simulink model "MGDC_RL"  (R2025b)
settings: Solver=VariableStepAuto  StartTime=0.0  StopTime=12  RelTol=1e-3
libraries: spsGroundLib x8, spsControlledVoltageSourceLib x3, spsCurrentMeasurementLib x3, spsParallelRLCBranchLib x3, spsVoltageMeasurementLib x3, spsSeriesRLCBranchLib x2, spsBreakerLib x1, sps_lib x1
(part 1 of 4)
settings Model: Creator=joseA  LastModifiedBy=joseA

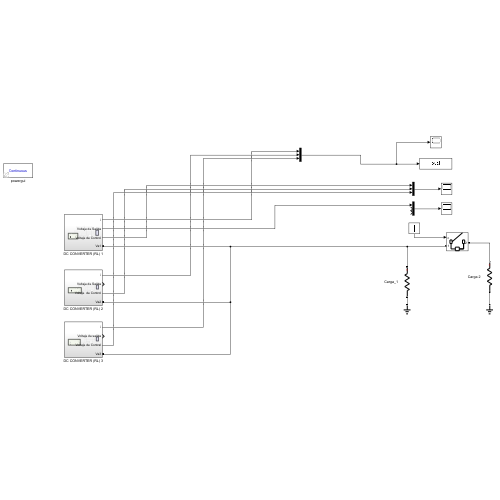
[thumbnail: Simulink's stored preview of the top-level diagram]
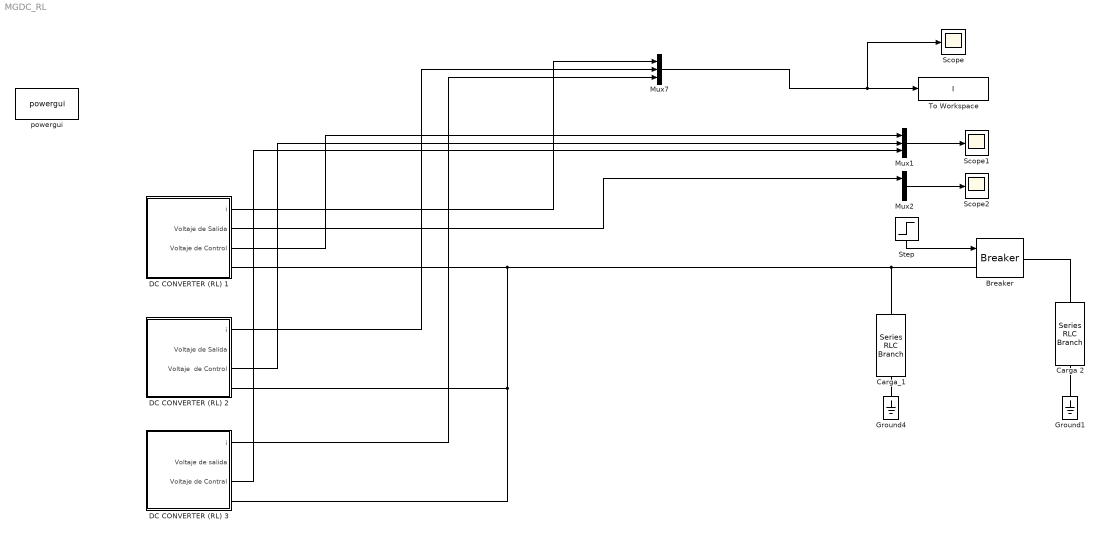
== system MGDC_RL ==
  Breaker : spsBreakerLib/Breaker  InitialState=0  SwitchingTimes="[1/60  5/60]"  External=on  BreakerResistance=0.01  SnubberResistance=1e6  SnubberCapacitance=inf  Measurements=None  MoreParameters=on  NoBreakLoop=off
  Carga 2 : spsSeriesRLCBranchLib/Series RLC Branch  LConnTagsString=__new0  RConnTagsString=__new0  BranchType=R  Resistance=4  Inductance=1e-3  SetiL0=off  InitialCurrent=0  Capacitance=1e-6  Setx0=off  InitialVoltage=0  Measurements=None
  Carga_1 : spsSeriesRLCBranchLib/Series RLC Branch  LConnTagsString=__new0  RConnTagsString=__new0  BranchType=R  Resistance=8  Inductance=1e-3  SetiL0=off  InitialCurrent=0  Capacitance=1e-6  Setx0=off  InitialVoltage=0  Measurements=None
  DC CONVERTER (RL) 1 : Subsystem
      settings: PortSchema="{\"entries\":[{\"content\":{\"sides\":[{\"content\":{\"connectorIds\":[\"Out1\",\"Out2\",\"Out3\",\"LConn1\"]},\"type\":\"ConnectorPlacement.EquallySpacedRectSide\",\"uuid\":\"ef85fad9-e9fc-446c-84f1-0628c69dc682\"},{\"content\":{\"side\":\"RIGHT\"},\"type\":\"ConnectorPlacement.EquallySpacedRectSide\",\"uuid\":\"b40e7fcd-3dee-4863-8a64-1e7c5a18af7f\"},{\"content\":{\"side\":\"TOP\"},\"type\":\"ConnectorPlacement.EquallySpacedRectSide\",\"uuid\":\"d80d7a5f-fa61-4dc2-bf12-1a6ce1f92f0b\"}]},\"type\":\"ConnectorPlacement.EquallySpacedConnector\",\"uuid\":\"ea08e065-469c-42e9-9976-17e3ee08db16\"}],\"packageUris\":[\"http://schema.mathworks.com/mf0/Connector/R2020b\"],\"version\":\"1.0\"}"
  DC CONVERTER (RL) 2 : Subsystem
      settings: PortSchema="{\"entries\":[{\"content\":{\"sides\":[{\"content\":{\"connectorIds\":[\"Out1\",\"Out2\",\"Out3\",\"LConn1\"]},\"type\":\"ConnectorPlacement.EquallySpacedRectSide\",\"uuid\":\"ef85fad9-e9fc-446c-84f1-0628c69dc682\"},{\"content\":{\"side\":\"RIGHT\"},\"type\":\"ConnectorPlacement.EquallySpacedRectSide\",\"uuid\":\"b40e7fcd-3dee-4863-8a64-1e7c5a18af7f\"},{\"content\":{\"side\":\"TOP\"},\"type\":\"ConnectorPlacement.EquallySpacedRectSide\",\"uuid\":\"d80d7a5f-fa61-4dc2-bf12-1a6ce1f92f0b\"}]},\"type\":\"ConnectorPlacement.EquallySpacedConnector\",\"uuid\":\"ea08e065-469c-42e9-9976-17e3ee08db16\"}],\"packageUris\":[\"http://schema.mathworks.com/mf0/Connector/R2020b\"],\"version\":\"1.0\"}"
  DC CONVERTER (RL) 3 : Subsystem
      settings: PortSchema="{\"entries\":[{\"content\":{\"sides\":[{\"content\":{\"connectorIds\":[\"Out1\",\"Out2\",\"Out3\",\"LConn1\"]},\"type\":\"ConnectorPlacement.EquallySpacedRectSide\",\"uuid\":\"ef85fad9-e9fc-446c-84f1-0628c69dc682\"},{\"content\":{\"side\":\"RIGHT\"},\"type\":\"ConnectorPlacement.EquallySpacedRectSide\",\"uuid\":\"b40e7fcd-3dee-4863-8a64-1e7c5a18af7f\"},{\"content\":{\"side\":\"TOP\"},\"type\":\"ConnectorPlacement.EquallySpacedRectSide\",\"uuid\":\"d80d7a5f-fa61-4dc2-bf12-1a6ce1f92f0b\"}]},\"type\":\"ConnectorPlacement.EquallySpacedConnector\",\"uuid\":\"ea08e065-469c-42e9-9976-17e3ee08db16\"}],\"packageUris\":[\"http://schema.mathworks.com/mf0/Connector/R2020b\"],\"version\":\"1.0\"}"
  Ground1 : spsGroundLib/Ground  LConnTagsString=a
  Ground4 : spsGroundLib/Ground  LConnTagsString=a
  Mux1 : Mux  Inputs=3
  Mux2 : Mux  Inputs=3
  Mux7 : Mux  Inputs=3
  Scope : Scope
      settings: ActiveDisplayYMinimum=-0.5913391401684992  ActiveDisplayYMaximum=5.3220510444351152
  Scope1 : Scope
      settings: ActiveDisplayYMinimum=-0.069374999999999867  ActiveDisplayYMaximum=0.67437499999999884
  Scope2 : Scope
      settings: ActiveDisplayYMinimum=-3.0088602206152393  ActiveDisplayYMaximum=27.079741985537161  DataLoggingVariableName=ScopeData3
  Step : Step  Time=6.5  SampleTime=0
  To Workspace : ToWorkspace  VariableName=I  SaveFormat=Timeseries  SampleTime=-1
  powergui : sps_lib/powergui  Priority=1  SimulationMode=Continuous  SampleTime=50e-6  frequency=60  Iterations=50  frequencyindice=0  Pbase=100e6  ErrMax=1e-4  UnitsV=kV  UnitsW=MW  buscounter=0  FunctionMessages=off  echomessages=off  EnableUseOfTLC=off  CurrentSourceSwitches=off  DisableSnubberDevices=off  DisableRonSwitches=off  DisableVfSwitches=off  DisplayEquations=off  AutomaticDiscreteSolvers=off  SolverType=Tustin/Backward Euler (TBE)  Interpol=off  ExternalGateDelay=off  methode=off  Ts=100  x0status=blocks  SPID=on  SwTol=0  HookPort=off  NonlinearTolerance=1e-4  nMaxIteration=100  ContinueOnMaxIteration=off  RestoreLinks=warning  ResistiveCurrentMeasurement=off  Frange=[0:2:500]  Ylog=off  Xlog=on  ShowGrid=off  save=off  variable=ZData  structure=0  ZoomFFT=off  StartTime=0.0  cycles=1  DisplayStyle=1  fundamental=60  FreqAxis=off  MaxFrequency=1000  frequencyindicesteady=1  RmsSteady=1  display=off
  wires:
  Step/1 -> Breaker/1
  DC CONVERTER (RL) 1/1(i) -> Mux7/1
  DC CONVERTER (RL) 3/1(i) -> Mux7/3
  Mux7/1 -> Scope/1, To Workspace/1
  DC CONVERTER (RL) 2/1(i) -> Mux7/2
  DC CONVERTER (RL) 1/3(Voltaje de Control) -> Mux1/1
  Mux1/1 -> Scope1/1
  DC CONVERTER (RL) 2/3(Voltaje  de Control) -> Mux1/2
  DC CONVERTER (RL) 3/3(Voltaje de Contral) -> Mux1/3
  DC CONVERTER (RL) 1/2(Voltaje de Salida) -> Mux2/1
  Mux2/1 -> Scope2/1
  connections:
  Ground1/LConn1 -- Carga 2/RConn1
  Ground4/LConn1 -- Carga_1/RConn1
  Carga 2/LConn1 -- Breaker/RConn1
  DC CONVERTER (RL) 2/LConn1 -- DC CONVERTER (RL) 3/LConn1 -- Breaker/LConn1 -- Carga_1/LConn1 -- DC CONVERTER (RL) 1/LConn1

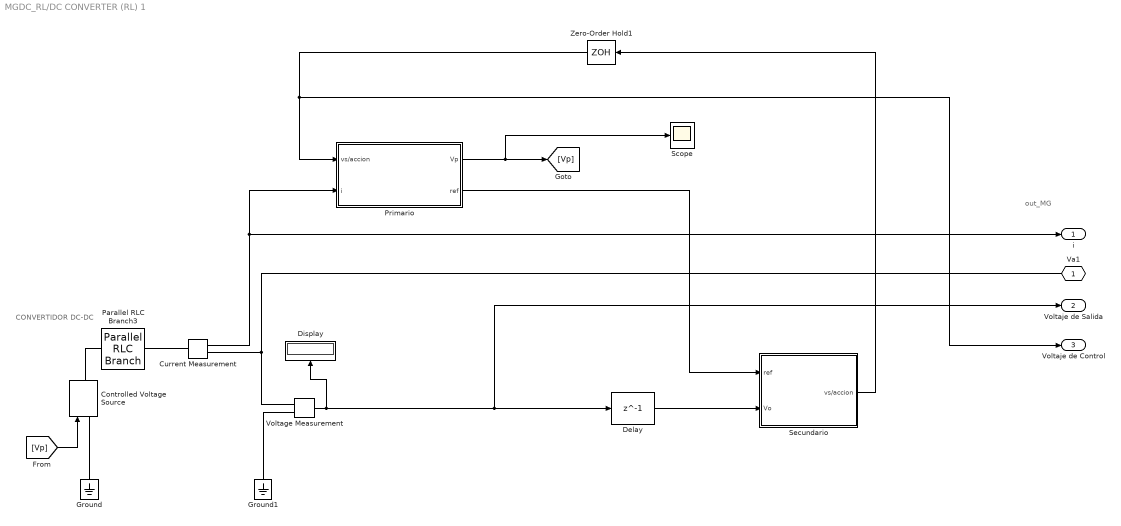
== system MGDC_RL/DC CONVERTER (RL) 1 ==
  note: out_MG
  note: CONVERTIDOR DC-DC
  Controlled Voltage Source : spsControlledVoltageSourceLib/Controlled Voltage Source  Initialize=on  Source_Type=DC  Amplitude=0  Phase=0  Frequency=0  Measurements=None
  Current Measurement : spsCurrentMeasurementLib/Current Measurement  PhasorSimulation=off  OutputType=Complex  PSBequivalent=0
  Delay : Delay  DelayLength=1  InitialCondition=0  UseCircularBuffer=on
  Display : Display
  Ground : spsGroundLib/Ground  LConnTagsString=a
  Ground1 : spsGroundLib/Ground  LConnTagsString=a
  Parallel RLC Branch3 : spsParallelRLCBranchLib/Parallel RLC Branch  LConnTagsString=a  RConnTagsString=__new0  BranchType=R  Resistance=0.01  Inductance=1e-3  SetiL0=off  InitialCurrent=0  Capacitance=1e-6  Setx0=off  InitialVoltage=0  Measurements=None
  Primario : Subsystem
  Scope : Scope
      settings: ActiveDisplayYMinimum=-1  ActiveDisplayYMaximum=1  DataLoggingVariableName=ScopeData2
  "Secundario " : Subsystem
  Voltage Measurement : spsVoltageMeasurementLib/Voltage Measurement  PhasorSimulation=off  OutputType=Complex  PSBequivalent=0
  Zero-Order Hold1 : ZeroOrderHold  SampleTime=0.01
  Va1 : PMIOPort  Tag=PMCPort  Side=Left
  i : Outport
  Voltaje de Salida : Outport  Port=2
  Voltaje de Control : Outport  Port=3
  wires:
  Voltage Measurement/1 -> Voltaje de Salida/1, Delay/1, Display/1
  [Vp] -> Controlled Voltage Source/1
  Zero-Order Hold1/1 -> Primario/1(vs/accion), Voltaje de Control/1
  Current Measurement/1 -> i/1, Primario/2(i)
  "Secundario "/1(vs/accion) -> Zero-Order Hold1/1
  Primario/2(ref) -> "Secundario "/1(ref)
  Delay/1 -> "Secundario "/2(Vo)
  Primario/1(Vp) -> Scope/1, [Vp]
  connections:
  Voltage Measurement/LConn2 -- Ground1/LConn1
  Ground/LConn1 -- Controlled Voltage Source/LConn1
  Parallel RLC Branch3/LConn1 -- Current Measurement/LConn1
  Voltage Measurement/LConn1 -- Va1/RConn1 -- Current Measurement/RConn1
  Controlled Voltage Source/RConn1 -- Parallel RLC Branch3/RConn1

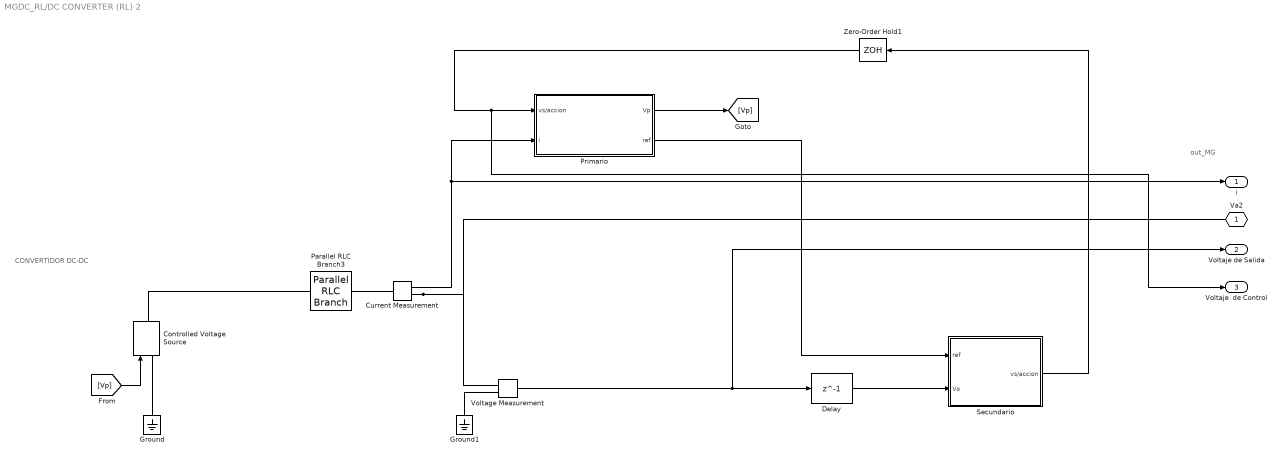
== system MGDC_RL/DC CONVERTER (RL) 2 ==
  note: out_MG
  note: CONVERTIDOR DC-DC
  Controlled Voltage Source : spsControlledVoltageSourceLib/Controlled Voltage Source  Initialize=on  Source_Type=DC  Amplitude=0  Phase=0  Frequency=0  Measurements=None
  Current Measurement : spsCurrentMeasurementLib/Current Measurement  PhasorSimulation=off  OutputType=Complex  PSBequivalent=0
  Delay : Delay  DelayLength=1  InitialCondition=0  UseCircularBuffer=on
  Ground : spsGroundLib/Ground  LConnTagsString=a
  Ground1 : spsGroundLib/Ground  LConnTagsString=a
  Parallel RLC Branch3 : spsParallelRLCBranchLib/Parallel RLC Branch  LConnTagsString=a  RConnTagsString=__new0  BranchType=R  Resistance=0.01  Inductance=1e-3  SetiL0=off  InitialCurrent=0  Capacitance=1e-6  Setx0=off  InitialVoltage=0  Measurements=None
  Primario : Subsystem
  "Secundario " : Subsystem
  Voltage Measurement : spsVoltageMeasurementLib/Voltage Measurement  PhasorSimulation=off  OutputType=Complex  PSBequivalent=0
  Zero-Order Hold1 : ZeroOrderHold  SampleTime=0.01
  Va2 : PMIOPort  Tag=PMCPort  Side=Left
  i : Outport
  Voltaje de Salida : Outport  Port=2
  Voltaje  de Control : Outport  Port=3
  wires:
  Voltage Measurement/1 -> Voltaje de Salida/1, Delay/1
  [Vp] -> Controlled Voltage Source/1
  Zero-Order Hold1/1 -> Voltaje  de Control/1, Primario/1(vs/accion)
  Current Measurement/1 -> i/1, Primario/2(i)
  "Secundario "/1(vs/accion) -> Zero-Order Hold1/1
  Primario/2(ref) -> "Secundario "/1(ref)
  Primario/1(Vp) -> [Vp]
  Delay/1 -> "Secundario "/2(Vo)
  connections:
  Voltage Measurement/LConn2 -- Ground1/LConn1
  Ground/LConn1 -- Controlled Voltage Source/LConn1
  Current Measurement/LConn1 -- Parallel RLC Branch3/LConn1
  Current Measurement/RConn1 -- Voltage Measurement/LConn1 -- Va2/RConn1
  Controlled Voltage Source/RConn1 -- Parallel RLC Branch3/RConn1

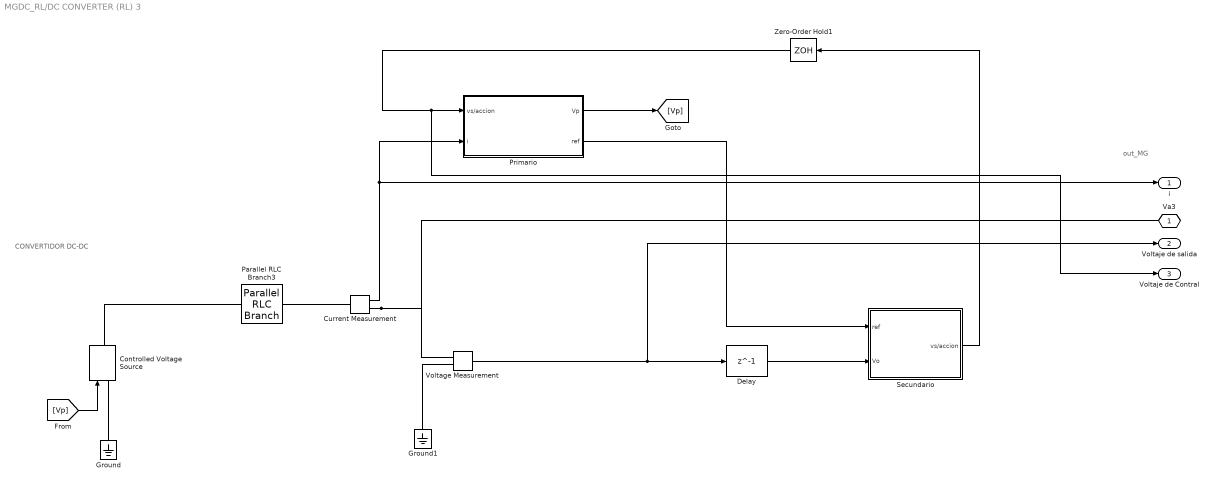
== system MGDC_RL/DC CONVERTER (RL) 3 ==
  note: out_MG
  note: CONVERTIDOR DC-DC
  Controlled Voltage Source : spsControlledVoltageSourceLib/Controlled Voltage Source  Initialize=on  Source_Type=DC  Amplitude=0  Phase=0  Frequency=0  Measurements=None
  Current Measurement : spsCurrentMeasurementLib/Current Measurement  PhasorSimulation=off  OutputType=Complex  PSBequivalent=0
  Delay : Delay  DelayLength=1  InitialCondition=0  UseCircularBuffer=on
  Ground : spsGroundLib/Ground  LConnTagsString=a
  Ground1 : spsGroundLib/Ground  LConnTagsString=a
  Parallel RLC Branch3 : spsParallelRLCBranchLib/Parallel RLC Branch  LConnTagsString=a  RConnTagsString=__new0  BranchType=R  Resistance=0.01  Inductance=1e-3  SetiL0=off  InitialCurrent=0  Capacitance=1e-6  Setx0=off  InitialVoltage=0  Measurements=None
  Primario : Subsystem
  "Secundario " : Subsystem
  Voltage Measurement : spsVoltageMeasurementLib/Voltage Measurement  PhasorSimulation=off  OutputType=Complex  PSBequivalent=0
  Zero-Order Hold1 : ZeroOrderHold  SampleTime=0.01
  Va3 : PMIOPort  Tag=PMCPort  Side=Left
  i : Outport
  Voltaje de salida : Outport  Port=2
  Voltaje de Contral : Outport  Port=3
  wires:
  Voltage Measurement/1 -> Voltaje de salida/1, Delay/1
  [Vp] -> Controlled Voltage Source/1
  Zero-Order Hold1/1 -> Voltaje de Contral/1, Primario/1(vs/accion)
  Current Measurement/1 -> i/1, Primario/2(i)
  "Secundario "/1(vs/accion) -> Zero-Order Hold1/1
  Primario/2(ref) -> "Secundario "/1(ref)
  Delay/1 -> "Secundario "/2(Vo)
  Primario/1(Vp) -> [Vp]
  connections:
  Voltage Measurement/LConn2 -- Ground1/LConn1
  Ground/LConn1 -- Controlled Voltage Source/LConn1
  Current Measurement/LConn1 -- Parallel RLC Branch3/LConn1
  Current Measurement/RConn1 -- Voltage Measurement/LConn1 -- Va3/RConn1
  Controlled Voltage Source/RConn1 -- Parallel RLC Branch3/RConn1

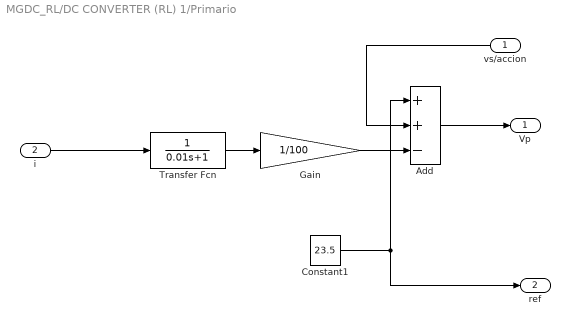
== system MGDC_RL/DC CONVERTER (RL) 1/Primario ==
  vs/accion : Inport
  i : Inport  Port=2
  Add : Sum  Inputs=++-
  Constant1 : Constant  Value=23.5
  Gain : Gain  Gain=1/100
  Transfer Fcn : TransferFcn  Denominator=[0.01 1]
  Vp : Outport
  ref : Outport  Port=2
  wires:
  vs/accion/1 -> Add/2
  Transfer Fcn/1 -> Gain/1
  Add/1 -> Vp/1
  Constant1/1 -> Add/1, ref/1
  Gain/1 -> Add/3
  i/1 -> Transfer Fcn/1

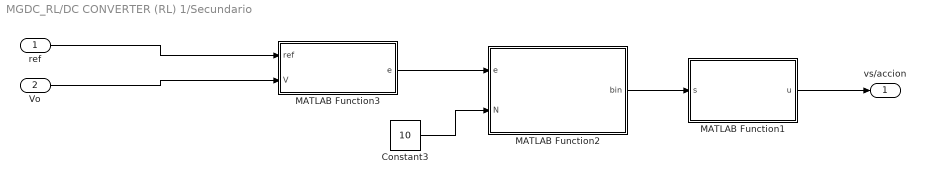
== system MGDC_RL/DC CONVERTER (RL) 1/Secundario  ==
  ref : Inport
  Vo : Inport  Port=2
  Constant3 : Constant  Value=10
  MATLAB Function1 : MATLAB Function  TreatAsAtomicUnit=on
  MATLAB Function2 : MATLAB Function  TreatAsAtomicUnit=on
  MATLAB Function3 : MATLAB Function  TreatAsAtomicUnit=on
  vs/accion : Outport
  wires:
  ref/1 -> MATLAB Function3/1(ref)
  Constant3/1 -> MATLAB Function2/2(N)
  MATLAB Function2/1(bin) -> MATLAB Function1/1(s)
  Vo/1 -> MATLAB Function3/2(V)
  MATLAB Function3/1(e) -> MATLAB Function2/1(e)
  MATLAB Function1/1(u) -> vs/accion/1

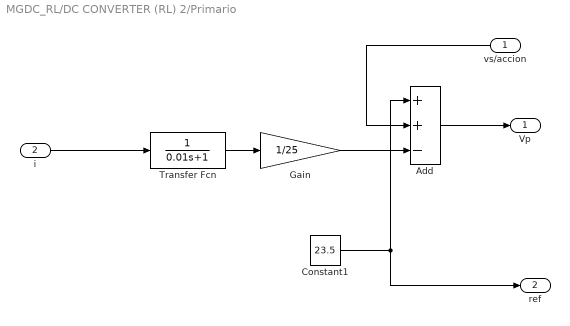
== system MGDC_RL/DC CONVERTER (RL) 2/Primario ==
  vs/accion : Inport
  i : Inport  Port=2
  Add : Sum  Inputs=++-
  Constant1 : Constant  Value=23.5
  Gain : Gain  Gain=1/25
  Transfer Fcn : TransferFcn  Denominator=[0.01 1]
  Vp : Outport
  ref : Outport  Port=2
  wires:
  vs/accion/1 -> Add/2
  Transfer Fcn/1 -> Gain/1
  Add/1 -> Vp/1
  Constant1/1 -> Add/1, ref/1
  Gain/1 -> Add/3
  i/1 -> Transfer Fcn/1

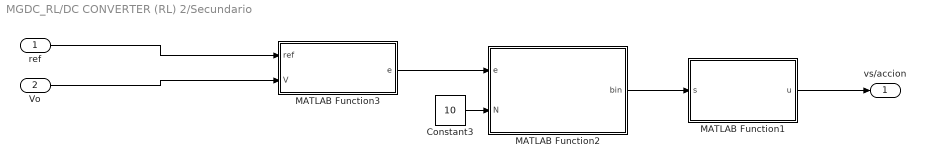
== system MGDC_RL/DC CONVERTER (RL) 2/Secundario  ==
  ref : Inport
  Vo : Inport  Port=2
  Constant3 : Constant  Value=10
  MATLAB Function1 : MATLAB Function  TreatAsAtomicUnit=on
  MATLAB Function2 : MATLAB Function  TreatAsAtomicUnit=on
  MATLAB Function3 : MATLAB Function  TreatAsAtomicUnit=on
  vs/accion : Outport
  wires:
  ref/1 -> MATLAB Function3/1(ref)
  Constant3/1 -> MATLAB Function2/2(N)
  MATLAB Function2/1(bin) -> MATLAB Function1/1(s)
  Vo/1 -> MATLAB Function3/2(V)
  MATLAB Function3/1(e) -> MATLAB Function2/1(e)
  MATLAB Function1/1(u) -> vs/accion/1

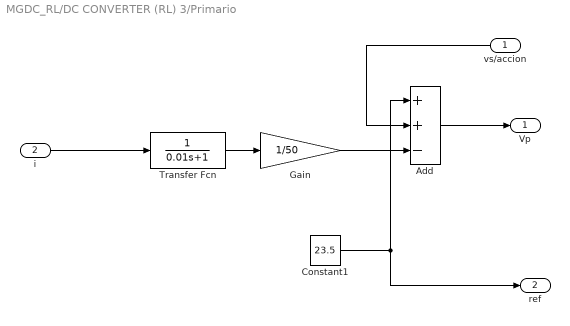
== system MGDC_RL/DC CONVERTER (RL) 3/Primario ==
  vs/accion : Inport
  i : Inport  Port=2
  Add : Sum  Inputs=++-
  Constant1 : Constant  Value=23.5
  Gain : Gain  Gain=1/50
  Transfer Fcn : TransferFcn  Denominator=[0.01 1]
  Vp : Outport
  ref : Outport  Port=2
  wires:
  vs/accion/1 -> Add/2
  Transfer Fcn/1 -> Gain/1
  Add/1 -> Vp/1
  Constant1/1 -> Add/1, ref/1
  Gain/1 -> Add/3
  i/1 -> Transfer Fcn/1

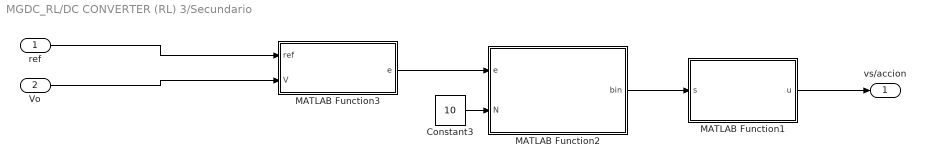
== system MGDC_RL/DC CONVERTER (RL) 3/Secundario  ==
  ref : Inport
  Vo : Inport  Port=2
  Constant3 : Constant  Value=10
  MATLAB Function1 : MATLAB Function  TreatAsAtomicUnit=on
  MATLAB Function2 : MATLAB Function  TreatAsAtomicUnit=on
  MATLAB Function3 : MATLAB Function  TreatAsAtomicUnit=on
  vs/accion : Outport
  wires:
  ref/1 -> MATLAB Function3/1(ref)
  Constant3/1 -> MATLAB Function2/2(N)
  MATLAB Function2/1(bin) -> MATLAB Function1/1(s)
  Vo/1 -> MATLAB Function3/2(V)
  MATLAB Function3/1(e) -> MATLAB Function2/1(e)
  MATLAB Function1/1(u) -> vs/accion/1
